simulink model "Q2_Control_Model"  (R2016b)
settings: Solver=VariableStepAuto  StartTime=0.0  StopTime=10.0  RelTol=1e-3
values from neighbouring files (symbols this model uses):
  J = 0.07    [CSD_HW_1_Script.m]
  K_t = 0.46    [CSD_HW_1_Script.m]
  N = 3    [CSD_HW_1_Script.m]    (also in Plotshit.m)
  R = 0.1    [CSD_HW_1_Script.m]    (also in Plotshit.m)
undefined symbols (not defined in the file or in its folder): K_e
settings Model: Creator=nadav  LastModifiedBy=nadav

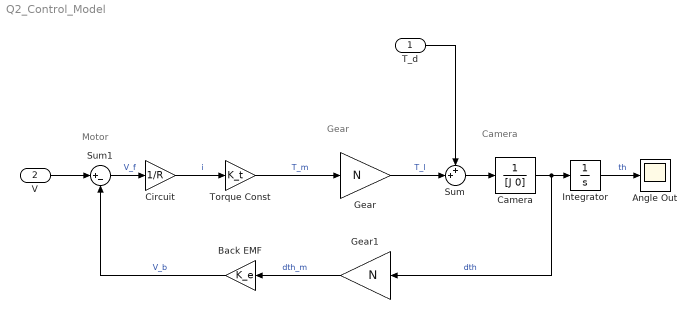
== system Q2_Control_Model ==
  note: Camera
  note: Gear
  note: Motor
  T_d : Inport
  V : Inport  Port=2
  Angle Out : Scope
  Back EMF : Gain  Gain=K_e
  Camera : TransferFcn  Denominator=[J 0]
  Circuit : Gain  Gain=1/R
  Gear : Gain  Gain=N
  Gear1 : Gain  Gain=N
  Integrator : Integrator
  Sum : Sum  Inputs=++|
  Sum1 : Sum  Inputs=|+-
  Torque Const : Gain  Gain=K_t
  wires:
  Gear/1 -> Sum/2  "T_l"
  Torque Const/1 -> Gear/1  "T_m"
  Circuit/1 -> Torque Const/1  "i"
  Gear1/1 -> Back EMF/1  "dth_m"
  Back EMF/1 -> Sum1/2  "V_b"
  Sum1/1 -> Circuit/1  "V_f"
  Integrator/1 -> Angle Out/1  "th"
  V/1 -> Sum1/1
  Sum/1 -> Camera/1
  Camera/1 -> Gear1/1, Integrator/1  "dth"
  T_d/1 -> Sum/1
